simulink model "project_model_part3_replyattack_detector2"  (R2020a)
settings: Solver=VariableStepAuto  StartTime=0.0  StopTime=130  RelTol=1e-3
undefined symbols (not defined in the file or in its folder): Discrete, Time
libraries: ctrlSharedLib x1
settings Model: Creator=Admin  LastModifiedBy=Shreya
settings DataIOCC: ReturnWorkspaceOutputs=off
settings DebuggingCC: ArithmeticOperatorsInVariantConditions=warning
settings SFSimCC: SimUseLocalCustomCode=off  CustomCodeUndefinedFunction=UseInterfaceOnly
settings RTWCC: RTWUseLocalCustomCode=off

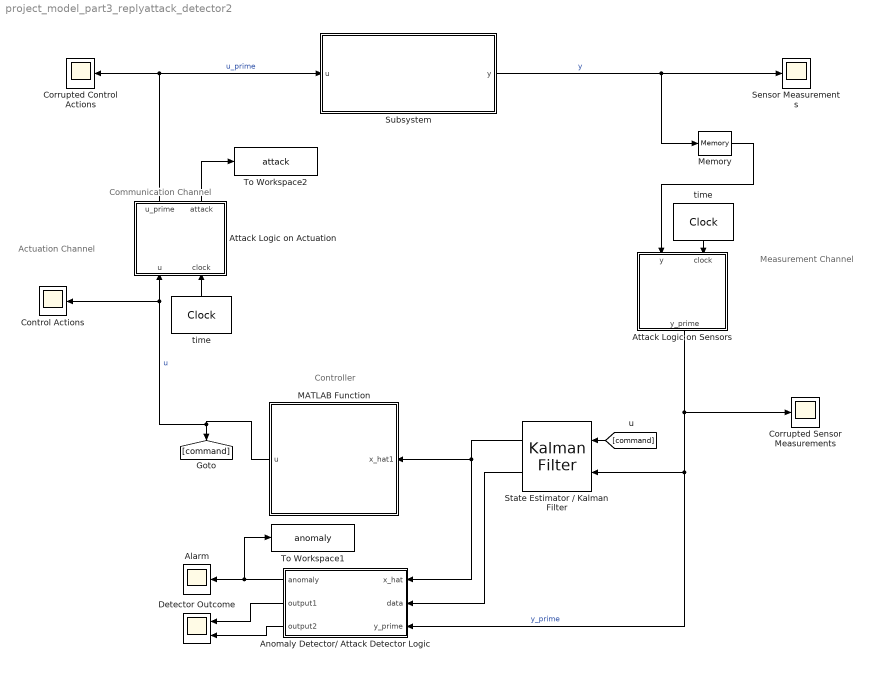
== system project_model_part3_replyattack_detector2 ==
  note: Controller
  note: Communication Channel
  note: Measurement Channel
  note: Actuation Channel
  Alarm : Scope
  Anomaly Detector/ Attack Detector Logic : MATLAB Function  TreatAsAtomicUnit=on
  Attack Logic on Actuation : MATLAB Function  TreatAsAtomicUnit=on
  Attack Logic on Sensors : MATLAB Function  TreatAsAtomicUnit=on
  Control Actions : Scope
  Corrupted Control Actions : Scope
  Corrupted Sensor Measurements : Scope
  Detector Outcome : Scope  NumInputPorts=2
  MATLAB Function : MATLAB Function  TreatAsAtomicUnit=on
  Memory : Memory  InitialCondition=-1  InheritSampleTime=on  LinearizeAsDelay=on
  "Sensor Measurements " : Scope
  State Estimator / Kalman Filter : ctrlSharedLib/Kalman Filter  TimeDomain=Discrete-Time  UseCurrentEstimator=on  ModelSource=Individual A, B, C, D matrices  ModelSourceVariable=sys  A="[1.0000    0.0001   -0.0010;0.5747    1.0000   -0.0003;0.0162    0.0000    1.0000]"  B="[0.1   -0.2; -0.0536    0.0332;0.1955   -0.5294];"  C=[1 0 0;0 1 0]  D=[0 0;0 0]  NumberOfStates=2  NumberOfInputs=2  NumberOfOutputs=2  InitialEstimateSource=Dialog  X0=[0;0;0]  P0=10  UseK=off  UseGH=off  NumberOfProcessNoiseInputs=2  G=1  TimeInvariantG=on  H=0  TimeInvariantH=on  Q=0.00001*eye(3)  TimeInvariantQ=on  R=0.00008*eye(2)  TimeInvariantR=on  N=0  TimeInvariantN=on  AddInputPort=on  AddEnablePort=off  OutputEstimatedY=off  OutputP=on  Ts=-1
  Subsystem : Subsystem
  To Workspace1 : ToWorkspace  VariableName=anomaly  SaveFormat=Timeseries  SampleTime=0.1
      settings: Save2DSignal=2-D array (concatenate along first dimension)
  To Workspace2 : ToWorkspace  VariableName=attack  SaveFormat=Timeseries  SampleTime=0.1
      settings: Save2DSignal=2-D array (concatenate along first dimension)
  time : DigitalClock  SampleTime=0.1
  "time " : DigitalClock  SampleTime=0.1
  wires:
  Anomaly Detector/ Attack Detector Logic/1(anomaly) -> To Workspace1/1, Alarm/1
  "time "/1 -> Attack Logic on Sensors/2(clock)
  Attack Logic on Sensors/1(y_prime) -> Anomaly Detector/ Attack Detector Logic/3(y_prime), State Estimator / Kalman Filter/2, Corrupted Sensor Measurements/1  "y_prime"
  MATLAB Function/1(u) -> Control Actions/1, Attack Logic on Actuation/1(u), [command]  "u"
  time/1 -> Attack Logic on Actuation/2(clock)
  Attack Logic on Actuation/1(u_prime) -> Subsystem/1(u), Corrupted Control Actions/1  "u_prime"
  [command] -> State Estimator / Kalman Filter/1
  Subsystem/1(y) -> Memory/1, "Sensor Measurements "/1  "y"
  State Estimator / Kalman Filter/1 -> MATLAB Function/1(x_hat1), Anomaly Detector/ Attack Detector Logic/1(x_hat)
  Memory/1 -> Attack Logic on Sensors/1(y)
  Anomaly Detector/ Attack Detector Logic/2(output1) -> Detector Outcome/1
  Anomaly Detector/ Attack Detector Logic/3(output2) -> Detector Outcome/2
  Attack Logic on Actuation/2(attack) -> To Workspace2/1
  State Estimator / Kalman Filter/2 -> Anomaly Detector/ Attack Detector Logic/2(data)

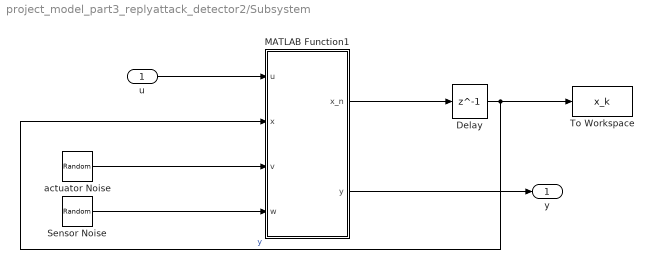
== system project_model_part3_replyattack_detector2/Subsystem ==
  u : Inport
  Delay : Delay  DelayLength=1  InitialCondition=[0 0.1 0.2]
  MATLAB Function1 : MATLAB Function  TreatAsAtomicUnit=on
  Sensor Noise : RandomNumber  Mean=[0 0]  Variance=[0.00008 0.00008]  Seed=[randi(100) randi(100)]
  To Workspace : ToWorkspace  VariableName=x_k  SaveFormat=Timeseries  SampleTime=-1
  actuator Noise : RandomNumber  Mean=[0 0 0]  Variance=[0.00001 0.00001 0.00001]  Seed=[randi(100) randi(100) randi(100)]
  y : Outport  VectorParamsAs1DForOutWhenUnconnected=off
  wires:
  u/1 -> MATLAB Function1/1(u)
  MATLAB Function1/1(x_n) -> Delay/1
  MATLAB Function1/2(y) -> y/1
  Sensor Noise/1 -> MATLAB Function1/4(w)
  actuator Noise/1 -> MATLAB Function1/3(v)
  Delay/1 -> To Workspace/1, MATLAB Function1/2(x)  "y"

== matlab function project_model_part3_replyattack_detector2/Attack Logic on Sensors ==
  data: y input; y_prime output; clock input
function y_prime = fcn(y,clock)
% this function should contain the attacker action on the sensor
% measurements
%Replay Attack Logic
y_prime = y;
persistent i
persistent j
persistent n
if isempty(i)
    i = 1;
end
if isempty(j)
    j = 1;
end
if isempty(n)
    n = zeros(200,2); 
end
if clock >= 80 && clock < 100
    %Data recored between 80 to 100 
    n(i,:) = transpose(y);
    i = i+1;  
elseif clock >= 100 && clock < 120 
    %Replay output between 100 to 120 
    y_prime = transpose(n(j,:));
    j = j+1;
else
   y_prime = y;
end
end

== matlab function project_model_part3_replyattack_detector2/MATLAB Function ==
  data: x_hat1 input; u output
function u  = Controller(x_hat1)
%two tanks model 
    

%controller gain
K =[17.1291   -1.1789   -6.5335; -0.1248   -2.9385   -2.5082];
u=-K*(x_hat1);

== matlab function project_model_part3_replyattack_detector2/Attack Logic on Actuation ==
  data: u input; u_prime output; clock input; attack output
function [u_prime,attack] = fcn(u,clock)
% this function should contain the attacker action on the control inputs
% Here u_a indicate false data vector 
if 0 <= clock && clock < 100
    u_a = transpose([0,0]);
    attack = 0;
elseif 100 <= clock && clock < 120
    u_a = transpose([-0.05 ,-0.05]);
    attack = 1;
else 
    u_a = transpose([0,0]);
    attack = 0;
end
u_prime = u + u_a;
end

== matlab function project_model_part3_replyattack_detector2/Anomaly Detector// Attack Detector Logic ==
  data: x_hat input; anomaly output; output1 output; output2 output; data input; y_prime input
function [anomaly,output1,output2] = Detector(x_hat,data,y_prime)
% this function should contain the detection strategy

% CUSUM detector logic
C = [1 0 0; 0 1 0];
R = 0.00008*eye(2);
%Here P is error covarience.
P = data;
sigma = (C * P * (transpose(C))) + R;
r = y_prime - (C * x_hat);
% Choosen Distance Measure but it is possible to drive CUSUM with any other distance measure
z = transpose(r) * (inv(sigma) * r);
%Here b is 'bias parameter'. For the tightest detection b is similar to P(state estimater error Covarience)
%Since z >= 0, the bias parameter b prevents the inherent growth due to the sum of nonnegative number.
%bias b must be selected properly based on the properties of the distance measure.
b = 2;
persistent s;
if isempty(s)
    %intially Cumulative sum is zero
    s = 0;
end
%Here beta is threshold value. 
%Once the bias is chosen, the threshold bita must be selected to fulfill a required false alarm rate.
beta = 13.5;
if s <= beta
    s = max([0,s + z - b]);
    output = 0;
    anomaly =0;
else
    s = 0;
    output = 1;
    anomaly = 1;
end
output1 = s;
output2 = beta;
end

== matlab function project_model_part3_replyattack_detector2/Subsystem/MATLAB Function1 ==
  data: x_n output; u input; y output; x input; v input; w input
function [x_n, y] = fcn(u, x, v, w)

A=[1.0000    0.0001   -0.0010;0.5747    1.0000   -0.0003;0.0162    0.0000    1.0000];
B = [0.1   -0.2; -0.0536    0.0332;0.1955   -0.5294];

C=[1 0 0;0 1 0];
D=[0 0;0 0];


x_n = A*x + B*u + v;
y = C*x + D*u + w;
